simulink subsystem "subG"  (R2022a)
settings: Solver=VariableStepAuto  StartTime=0.0  StopTime=10.0  RelTol=1e-3
settings Model: Creator=dileepan  LastModifiedBy=dileepan

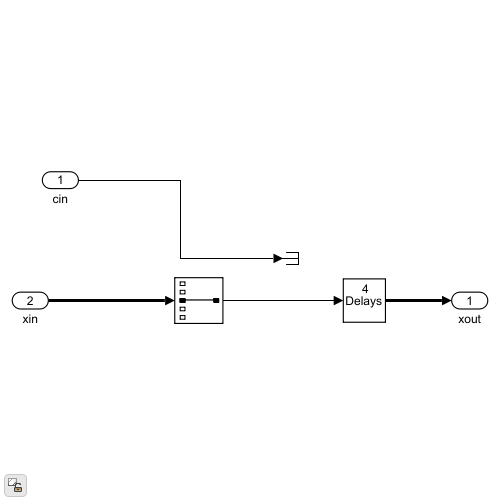
[thumbnail: Simulink's stored preview of the top-level diagram]
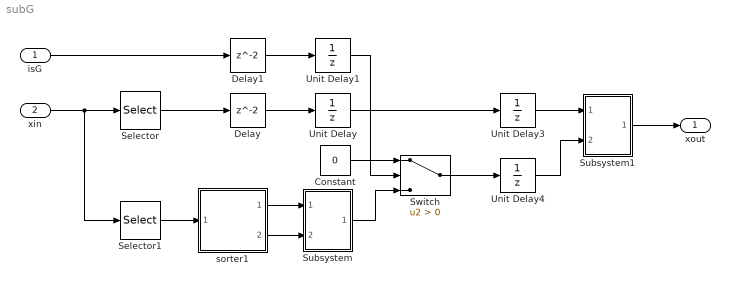
== system subG ==
  isG : Inport
  xin : Inport  Port=2
  Constant : Constant  Value=0  OutDataTypeStr=Inherit: Inherit via back propagation
  Delay : Delay
  Delay1 : Delay
  Selector : Selector  InputPortWidth=5  IndexOptions=Index vector (dialog)  Indices=3  OutputSizes=1
  Selector1 : Selector  InputPortWidth=5  IndexOptions=Index vector (dialog)  Indices=[1:2 4:5]  OutputSizes=1
  Subsystem : Subsystem  TreatAsAtomicUnit=on  ReferencedSubsystem=mean2
  Subsystem1 : Subsystem  TreatAsAtomicUnit=on  ReferencedSubsystem=sub2
  Switch : Switch  Criteria=u2 > Threshold  SaturateOnIntegerOverflow=off  InputSameDT=off
  Unit Delay{,1,3..4} (4 alike) : UnitDelay  SampleTime=-1  HasFrameUpgradeWarning=on
  sorter1 : Subsystem  TreatAsAtomicUnit=on  ReferencedSubsystem=median4
  xout : Outport
  wires:
  sorter1/1 -> Subsystem/1
  sorter1/2 -> Subsystem/2
  Selector1/1 -> sorter1/1
  xin/1 -> Selector1/1, Selector/1
  Selector/1 -> Delay/1
  Delay/1 -> Unit Delay/1
  Constant/1 -> Switch/1
  isG/1 -> Delay1/1
  Delay1/1 -> Unit Delay1/1
  Unit Delay1/1 -> Switch/2
  Subsystem1/1 -> xout/1
  Unit Delay/1 -> Unit Delay3/1
  Unit Delay3/1 -> Subsystem1/1
  Switch/1 -> Unit Delay4/1
  Subsystem/1 -> Switch/3
  Unit Delay4/1 -> Subsystem1/2
